simulink model "mcb_openloop_host"  (R2021a)
settings: Solver=FixedStepDiscrete  StartTime=0.0  StopTime=inf  RelTol=1e-3  EnableMultiTasking=on
libraries: mcbhostblockslib x3, simulink x3
settings Model: Creator=The MathWorks, Inc.  LastModifiedBy=Prasad Hegde
settings SolverCC: AlgebraicLoopSolver=TrustRegion
settings DataIOCC: LimitDataPoints=on  SaveFormat=Array  ReturnWorkspaceOutputs=off
settings OptimizationCC: LifeSpan=1  EfficientTunableParamExpr=on
settings DebuggingCC: MergeDetectMultiDrivingBlocksExec=none  SolverPrmCheckMsg=warning  ParameterPrecisionLossMsg=none  AllowSymbolicDim=off  PregeneratedLibrarySubsystemCodeDiagnostic=none  SFUnexpectedBacktrackingDiag=warning  SFNoUnconditionalDefaultTransitionDiag=warning  SFExecutionAtInitializationDiag=none  SFMachineParentedDataDiag=warning  ArithmeticOperatorsInVariantConditions=warning
settings HardwareCC: ProdBitPerPointer=32  ProdLargestAtomicFloat=None  ProdIntDivRoundTo=Undefined  ProdEndianess=Unspecified  ProdWordSize=32  ProdHWDeviceType=32-bit Generic
settings ModelReferenceCC: PropagateSignalLabelsOutOfModel=off
settings SFSimCC: SimUseLocalCustomCode=off  MATLABDynamicMemAlloc=off
settings RTWCC: Description=Real-Time Workshop Embedded Coder  SystemTargetFile=ert.tlc  TemplateMakefile=ert_default_tmf  GenerateReport=on  RTWUseLocalCustomCode=off  IncludeHyperlinkInReport=on  LaunchReport=on  GenerateTraceInfo=on  GenerateTraceReport=on  GenerateTraceReportSl=on  GenerateTraceReportSf=on  GenerateTraceReportEml=on
settings CodeAppCC: IgnoreCustomStorageClasses=off  StateflowObjectComments=on  InternalIdentifier=Classic
settings ERTTargetCC: MultiwordLength=2048  GenerateSampleERTMain=on  ERTCustomFileTemplate=example_file_process.tlc  ConvertIfToSwitch=off  SuppressUnreachableDefaultCases=off
settings ConfigComp: CovMetricSettings=dw  CovSaveCumulativeToWorkspaceVar=on  CovSaveSingleToWorkspaceVar=on  CovExternalEMLEnable=off  CovSFcnEnable=off

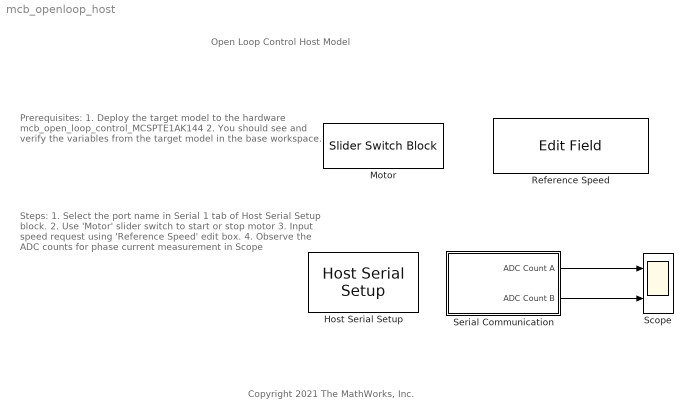
== system mcb_openloop_host ==
  note: Open Loop Control Host Model
  note: Steps:
      | 1. Select the port name in Serial 1 tab of
      | Host Serial Setup block.
      | 2. Use 'Motor' slider switch to start or stop motor
      | 3. Input speed request using 'Reference Speed'
      | edit box.
      | 4. Observe the ADC counts for phase current
      | measurement in Scope
  note: Prerequisites:
      | 1. Deploy the target model to the hardware
      | mcb_open_loop_control_MCSPTE1AK144
      |
      | 2. You should see and verify the variables
      | from the target model in the base
      | workspace.
  note: Copyright 2021 The MathWorks, Inc.
  Host Serial Setup : mcbhostblockslib/Host Serial Setup  Priority=-99  comPortSer1='Please_select_a_port'  baudRateA=256000  charLenA=8  stopBitA=1  parityA=none  timeoutA=2  ByteOrderA=LittleEndian  comPortSer2='Please_select_a_port'  baudRateB=115200  charLenB=8  stopBitB=1  parityB=none  timeoutB=1.0  ByteOrderB=LittleEndian  comPortSer3='Please_select_a_port'  baudRateC=115200  charLenC=8  stopBitC=1  parityC=none  timeoutC=1.0  ByteOrderC=LittleEndian  comPortSer4='Please_select_a_port'  baudRateD=115200  charLenD=8  stopBitD=1  parityD=none  timeoutD=1.0  ByteOrderD=LittleEndian
      settings: SourceProductBaseCode=MT
  Motor : SliderSwitchBlock  LabelPosition=Hide
      settings: Values={{'Stop', 'Start'}, [0 1]}
  Reference Speed : EditField  LabelPosition=Hide  ShowInitialText=on  Alignment=Center
  Scope : Scope  NumInputPorts=2
  Serial Communication : Subsystem
  wires:
  Serial Communication/1(ADC Count A) -> Scope/1
  Serial Communication/2(ADC Count B) -> Scope/2

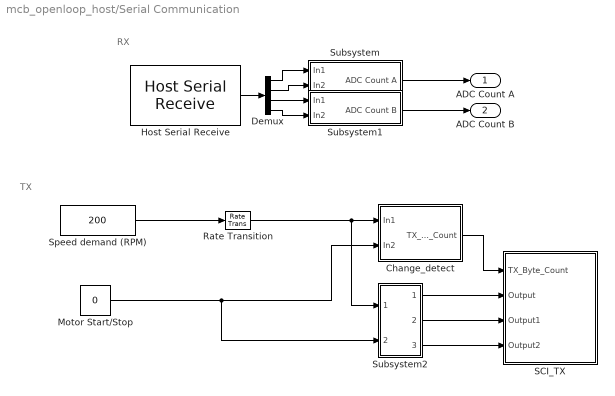
== system mcb_openloop_host/Serial Communication ==
  note: RX
  note: TX
  Change_detect : Subsystem
  Demux : Demux
  Host Serial Receive : mcbhostblockslib/Host Serial Receive  serialCon=Serial 1  dataHead='S'  dataTail='E'  dataType=uint8  dataDim=4  initValue=5  errOption=Output custom value  errValue=15  sampleTime=Ts_uart  outputStatus=off  blockingMode=on
      settings: SourceProductBaseCode=MT
  Motor Start/Stop : Constant  Value=0  OutDataTypeStr=Inherit: Inherit via back propagation
  Rate Transition : RateTransition  OutPortSampleTime=Ts_uart
  SCI_TX : Subsystem  TreatAsAtomicUnit=on
  Speed demand (RPM) : Constant  Value=200  VectorParams1D=off  OutDataTypeStr=int16  SampleTime=0.03
  Subsystem : Subsystem
  Subsystem1 : Subsystem
  Subsystem2 : Subsystem
  ADC Count A : Outport
  ADC Count B : Outport  Port=2
  wires:
  Motor Start/Stop/1 -> Subsystem2/2(In2), Change_detect/2(In2)
  Subsystem/1(ADC Count A) -> ADC Count A/1
  Subsystem1/1(ADC Count B) -> ADC Count B/1
  Rate Transition/1 -> Subsystem2/1(In1), Change_detect/1(In1)
  Host Serial Receive/1 -> Demux/1
  Demux/2 -> Subsystem/2(In2)
  Demux/1 -> Subsystem/1(In1)
  Demux/3 -> Subsystem1/1(In1)
  Demux/4 -> Subsystem1/2(In2)
  Speed demand (RPM)/1 -> Rate Transition/1
  Subsystem2/1(Output) -> SCI_TX/2(Output)
  Subsystem2/2(Output1) -> SCI_TX/3(Output1)
  Subsystem2/3(Output2) -> SCI_TX/4(Output2)
  Change_detect/1(TX_Byte_Count) -> SCI_TX/1(TX_Byte_Count)

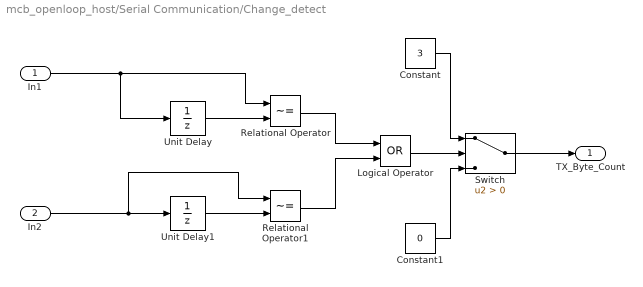
== system mcb_openloop_host/Serial Communication/Change_detect ==
  In1 : Inport
  In2 : Inport  Port=2
  Constant : Constant  Value=3  OutDataTypeStr=uint8
  Constant1 : Constant  Value=0  OutDataTypeStr=uint8
  Logical Operator : Logic  Operator=OR  AllPortsSameDT=off  OutDataTypeStr=boolean
  Relational Operator : RelationalOperator  Operator=~=  OutDataTypeStr=boolean  RndMeth=Nearest
  Relational Operator1 : RelationalOperator  Operator=~=  OutDataTypeStr=boolean  RndMeth=Nearest
  Switch : Switch  Criteria=u2 > Threshold
  Unit Delay : UnitDelay  InitialCondition=0.5  SampleTime=-1  HasFrameUpgradeWarning=on
  Unit Delay1 : UnitDelay  SampleTime=-1  HasFrameUpgradeWarning=on
  TX_Byte_Count : Outport  VectorParamsAs1DForOutWhenUnconnected=off
  wires:
  In2/1 -> Relational Operator1/1, Unit Delay1/1
  Unit Delay1/1 -> Relational Operator1/2
  Relational Operator1/1 -> Logical Operator/2
  Unit Delay/1 -> Relational Operator/2
  In1/1 -> Relational Operator/1, Unit Delay/1
  Relational Operator/1 -> Logical Operator/1
  Logical Operator/1 -> Switch/2
  Switch/1 -> TX_Byte_Count/1
  Constant/1 -> Switch/1
  Constant1/1 -> Switch/3

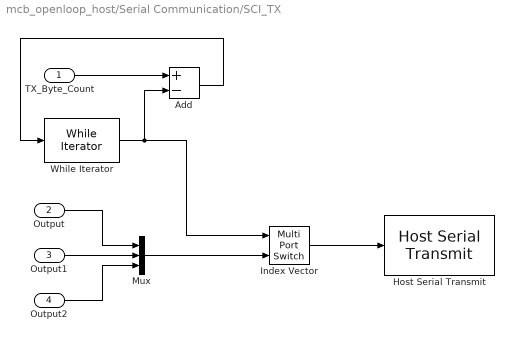
== system mcb_openloop_host/Serial Communication/SCI_TX ==
  TX_Byte_Count : Inport
  Output : Inport  Port=2
  Output1 : Inport  Port=3
  Output2 : Inport  Port=4
  Add : Sum  Inputs=+-  OutDataTypeStr=Inherit: Same as first input
  Host Serial Transmit : mcbhostblockslib/Host Serial Transmit  serialCon=Serial 1  header=''  tail=''  enableBlockingMode=off
      settings: SourceProductBaseCode=MT
  Index Vector : MultiPortSwitch  Inputs=1
  Mux : Mux  Inputs=3
  While Iterator : WhileIterator  MaxIters=3  WhileBlockType=do-while  ShowIterationPort=on  OutputDataType=int16
  wires:
  Output/1 -> Mux/1
  Mux/1 -> Index Vector/2
  Output2/1 -> Mux/3
  Add/1 -> While Iterator/1
  Output1/1 -> Mux/2
  TX_Byte_Count/1 -> Add/1
  While Iterator/1 -> Index Vector/1, Add/2
  Index Vector/1 -> Host Serial Transmit/1

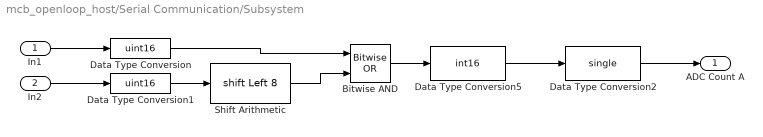
== system mcb_openloop_host/Serial Communication/Subsystem ==
  In1 : Inport
  In2 : Inport  Port=2
  Bitwise AND : simulink/Logic and Bit Operations/Bitwise Operator  logicop=OR  UseBitMask=off  NumInputPorts=2  BitMask=bin2dec('11011001')  BitMaskRealWorld=Stored Integer
  Data Type Conversion : DataTypeConversion  OutDataTypeStr=uint16  RndMeth=Simplest
  Data Type Conversion1 : DataTypeConversion  OutDataTypeStr=uint16  RndMeth=Simplest
  Data Type Conversion2 : DataTypeConversion  OutDataTypeStr=single  RndMeth=Simplest
  Data Type Conversion5 : DataTypeConversion  OutDataTypeStr=int16  ConvertRealWorld=Stored Integer (SI)  RndMeth=Simplest
  Shift Arithmetic : ArithShift  BitShiftNumber=8  BitShiftDirection=Left
  ADC Count A : Outport
  wires:
  In1/1 -> Data Type Conversion/1
  Data Type Conversion5/1 -> Data Type Conversion2/1
  In2/1 -> Data Type Conversion1/1
  Shift Arithmetic/1 -> Bitwise AND/2
  Bitwise AND/1 -> Data Type Conversion5/1
  Data Type Conversion1/1 -> Shift Arithmetic/1
  Data Type Conversion/1 -> Bitwise AND/1
  Data Type Conversion2/1 -> ADC Count A/1

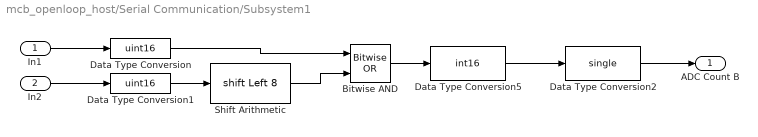
== system mcb_openloop_host/Serial Communication/Subsystem1 ==
  In1 : Inport
  In2 : Inport  Port=2
  Bitwise AND : simulink/Logic and Bit Operations/Bitwise Operator  logicop=OR  UseBitMask=off  NumInputPorts=2  BitMask=bin2dec('11011001')  BitMaskRealWorld=Stored Integer
  Data Type Conversion : DataTypeConversion  OutDataTypeStr=uint16  RndMeth=Simplest
  Data Type Conversion1 : DataTypeConversion  OutDataTypeStr=uint16  RndMeth=Simplest
  Data Type Conversion2 : DataTypeConversion  OutDataTypeStr=single  RndMeth=Simplest
  Data Type Conversion5 : DataTypeConversion  OutDataTypeStr=int16  ConvertRealWorld=Stored Integer (SI)  RndMeth=Simplest
  Shift Arithmetic : ArithShift  BitShiftNumber=8  BitShiftDirection=Left
  ADC Count B : Outport
  wires:
  Data Type Conversion/1 -> Bitwise AND/1
  Data Type Conversion1/1 -> Shift Arithmetic/1
  Bitwise AND/1 -> Data Type Conversion5/1
  Shift Arithmetic/1 -> Bitwise AND/2
  In2/1 -> Data Type Conversion1/1
  Data Type Conversion5/1 -> Data Type Conversion2/1
  In1/1 -> Data Type Conversion/1
  Data Type Conversion2/1 -> ADC Count B/1

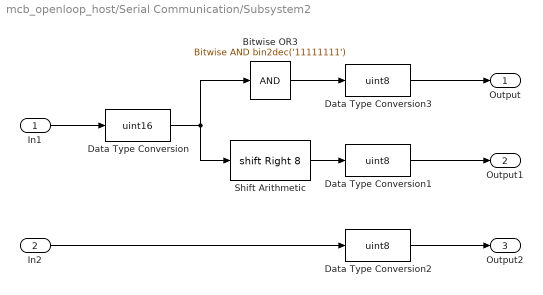
== system mcb_openloop_host/Serial Communication/Subsystem2 ==
  In1 : Inport
  In2 : Inport  Port=2
  Bitwise OR3 : simulink/Logic and Bit Operations/Bitwise Operator  logicop=AND  UseBitMask=on  BitMask=bin2dec('11111111')  BitMaskRealWorld=Stored Integer
  Data Type Conversion : DataTypeConversion  OutDataTypeStr=uint16  ConvertRealWorld=Stored Integer (SI)  RndMeth=Simplest
  Data Type Conversion1 : DataTypeConversion  OutDataTypeStr=uint8  ConvertRealWorld=Stored Integer (SI)  RndMeth=Simplest
  Data Type Conversion2 : DataTypeConversion  OutDataTypeStr=uint8  ConvertRealWorld=Stored Integer (SI)  RndMeth=Simplest
  Data Type Conversion3 : DataTypeConversion  OutDataTypeStr=uint8  ConvertRealWorld=Stored Integer (SI)  RndMeth=Simplest
  Shift Arithmetic : ArithShift  BitShiftNumber=8  BitShiftDirection=Right
  Output : Outport
  Output1 : Outport  Port=2
  Output2 : Outport  Port=3
  wires:
  Data Type Conversion2/1 -> Output2/1
  Data Type Conversion/1 -> Bitwise OR3/1, Shift Arithmetic/1
  In1/1 -> Data Type Conversion/1
  Bitwise OR3/1 -> Data Type Conversion3/1
  Shift Arithmetic/1 -> Data Type Conversion1/1
  In2/1 -> Data Type Conversion2/1
  Data Type Conversion1/1 -> Output1/1
  Data Type Conversion3/1 -> Output/1
